simulink model "time_delay_continuous_model"  (R2023b)
settings: Solver=VariableStepAuto  StartTime=0.0  StopTime=20  RelTol=1e-3
values from neighbouring files (symbols this model uses):
  A = [Aaa Aab; Aba Abb]    [compensated_minimum_order_controller.m]    (also in compensated_observer_controller.m = [A Bv*Cc; zeros(1, 3) Ac]; direct_comp_calib.m; direct_compensated_minimum_order_controller.m; experiment_calc.m)
  AA = [A-Bv*K Bv*(Kb-[0 1 0]*A_b*kc); zeros(2, 3) Ae-Ko*Aab]    [compensated_minimum_order_controller.m]    (also in compensated_observer_controller.m = [A-Bv*K Bv*K; zeros(4) A-Ke*C]; direct_comp_calib.m = [A-Bv*K Bv*Kb; zeros(2, 3) Abb-Ko*Aab]; direct_compensated_minimum_order_controller.m = [A-Bv*K Bv*Kb; zeros(2, 3) Abb-Ko*Aab]; experiment_calc.m = [A-Bv*K Bv*Kb; zeros([2, 3]) Abb - Ko*Aab])
  Ahat = Abb - Ko*Aab    [experiment_calc.m]    (also in experiment_sym.m; simple_time_delay_discrete.m; simple_time_delay_sym.m; time_delay_continuous.m)
  Aimp = [0 1; -Ke/Me -Be/Me]    [experiment_calc.m]    (also in experiment_sym.m; time_delay_continuous.m; time_delay_continuous_sym.m; time_delay_discrete.m)
  Atilde = Ahat - Fhat_v*Kb    [experiment_calc.m]    (also in experiment_sym.m; simple_time_delay_discrete.m = Ahat - Fhat*Kb; simple_time_delay_sym.m = Ahat - Fhat*Kb; time_delay_continuous.m)
  B = -8*P.*M*0.05    [comp_controller_param_map.m]    (also in compensated_minimum_order_controller.m = [Bt Bv]; compensated_observer_controller.m = [0 0; 1/J 0; 0 1/L]; direct_comp_calib.m = [Bt Bv]; direct_compensated_minimum_order_controller.m = [Bt Bv])
  BB = [Bt - Bv*kc; zeros(2, 1)]    [compensated_minimum_order_controller.m]    (also in compensated_observer_controller.m = [Bt; Bt]; direct_comp_calib.m; direct_compensated_minimum_order_controller.m; experiment_calc.m = [Bv*Ka Bt - Bv*kc; zeros([2, 2])])
  Bhat = Ahat*Ko + Aba - Ko*Aaa    [experiment_calc.m]    (also in experiment_sym.m; simple_time_delay_discrete.m; simple_time_delay_sym.m; time_delay_continuous.m)
  Bimp = [0 0; Ke/Me 1/Me]    [experiment_calc.m]    (also in experiment_sym.m; time_delay_continuous.m; time_delay_continuous_sym.m; time_delay_discrete.m)
  Btilde = [Btilde_r Btilde_tau Btilde_y]    [experiment_calc.m]    (also in experiment_sym.m; simple_time_delay_discrete.m = [Btilde_r Btilde_y]; simple_time_delay_sym.m = [Btilde_r Btilde_y]; time_delay_continuous.m)
  C = [1 0 0]    [compensated_minimum_order_controller.m]    (also in compensated_observer_controller.m = [C 0]; direct_comp_calib.m; direct_compensated_minimum_order_controller.m; experiment_calc.m)
  CC = eye(5)    [compensated_minimum_order_controller.m]    (also in compensated_observer_controller.m = eye(8); direct_comp_calib.m; direct_compensated_minimum_order_controller.m; experiment_calc.m)
  Chat = [zeros([1, 2]); eye(2)]    [experiment_calc.m]    (also in experiment_sym.m; simple_time_delay_discrete.m = [0; 1]; simple_time_delay_sym.m = [0; 1]; time_delay_continuous.m)
  Cimp = [1 0]    [experiment_calc.m]    (also in experiment_sym.m = eye(2); time_delay_continuous.m = eye(2); time_delay_continuous_sym.m; time_delay_discrete.m = eye(2))
  Ctilde = -Kb    [experiment_calc.m]    (also in experiment_sym.m; simple_time_delay_discrete.m; simple_time_delay_sym.m; time_delay_continuous.m)
  D = [0 0]    [compensated_minimum_order_controller.m]    (also in compensated_observer_controller.m = 0; direct_comp_calib.m; direct_compensated_minimum_order_controller.m; experiment_calc.m)
  DD = zeros(5, 1)    [compensated_minimum_order_controller.m]    (also in compensated_observer_controller.m = zeros(8, 1); direct_comp_calib.m; direct_compensated_minimum_order_controller.m; experiment_calc.m = zeros([5, 2]))
  Dhat = [1; Ko]    [experiment_calc.m]    (also in experiment_sym.m; simple_time_delay_discrete.m; simple_time_delay_sym.m; time_delay_continuous.m)
  Dimp = zeros(2)    [experiment_calc.m]    (also in experiment_sym.m; time_delay_continuous.m; time_delay_continuous_sym.m; time_delay_discrete.m)
  Dtilde = [Ka -kc -(Ka + Kb*Ko)]    [experiment_calc.m]    (also in experiment_sym.m; simple_time_delay_discrete.m = [Ka -(Ka + Kb*Ko)]; simple_time_delay_sym.m = [Ka -(Ka + Kb*Ko)]; time_delay_continuous.m)
  ei = [0; 0]    [experiment_sym.m]    (also in simple_time_delay_discrete.m = 0; time_delay_continuous.m; time_delay_discrete.m; time_delay_discrete_fourier.m)
  Fhat_tau = Btb - Ko*Bta    [experiment_calc.m]    (also in experiment_sym.m; time_delay_continuous.m; time_delay_continuous_sym.m; time_delay_discrete.m)
  Fhat_v = Bvb - Ko*Bva    [experiment_calc.m]    (also in experiment_sym.m; time_delay_continuous.m; time_delay_continuous_sym.m; time_delay_discrete.m)
  K = place(A, Bv, P)    [compensated_minimum_order_controller.m]    (also in compensated_observer_controller.m; direct_comp_calib.m = acker(A, Bv, P); direct_compensated_minimum_order_controller.m = acker(A, Bv, P); experiment_calc.m = [0 0 1]/Cm*pd)
  Ka = K(1)    [compensated_minimum_order_controller.m]    (also in direct_comp_calib.m; direct_compensated_minimum_order_controller.m; experiment_calc.m; experiment_sym.m)
  kc = (R+K(3))/Km-Ka/Ke    [compensated_minimum_order_controller.m]    (also in direct_comp_calib.m; direct_compensated_minimum_order_controller.m; experiment_calc.m; experiment_sym.m)
  nutildei = nui - ei    [experiment_sym.m]    (also in simple_time_delay_discrete.m; time_delay_continuous.m; time_delay_discrete.m)
  xi = [1; 0; 0]    [experiment_sym.m]    (also in simple_time_delay_discrete.m = [1; 0]; time_delay_continuous.m = [0; 0; 0]; time_delay_discrete.m = [0; 0; 0]; time_delay_discrete_fourier.m)
settings Model: Creator=tamas  LastModifiedBy=tamas

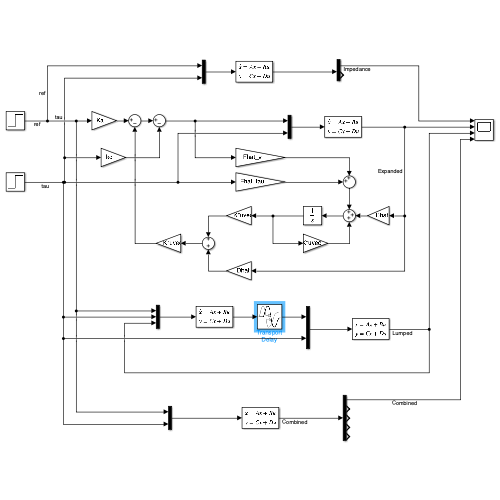
[thumbnail: Simulink's stored preview of the top-level diagram]
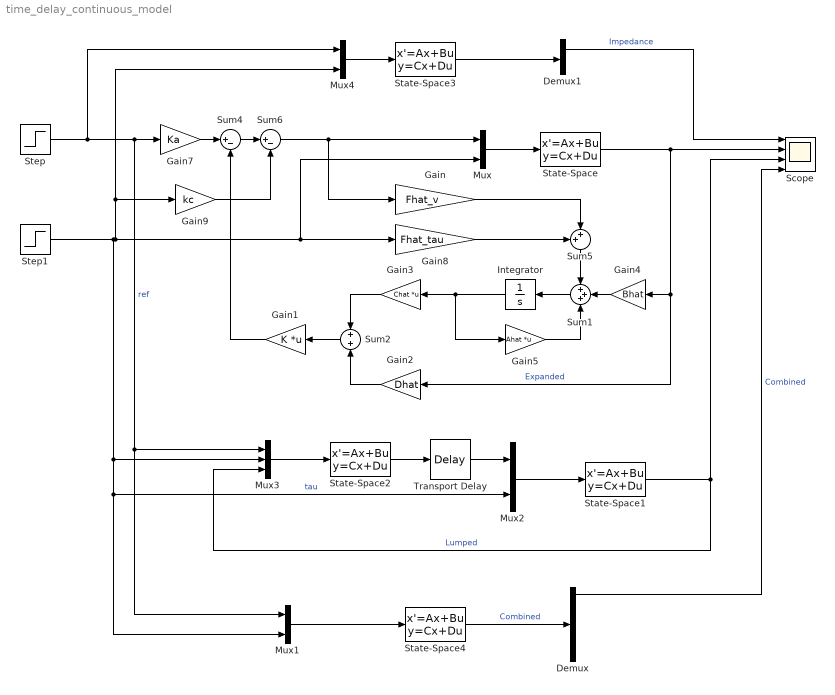
== system time_delay_continuous_model ==
  Demux : Demux  Outputs=5
  Demux1 : Demux  Outputs=2
  Gain : Gain  Gain=Fhat_v
  Gain1 : Gain  Gain=K  Multiplication=Matrix(K*u) (u vector)
  Gain2 : Gain  Gain=Dhat
  Gain3 : Gain  Gain=Chat  Multiplication=Matrix(K*u) (u vector)
  Gain4 : Gain  Gain=Bhat
  Gain5 : Gain  Gain=Ahat  Multiplication=Matrix(K*u) (u vector)
  Gain7 : Gain  Gain=Ka
  Gain8 : Gain  Gain=Fhat_tau
  Gain9 : Gain  Gain=kc
  Integrator : Integrator  InitialCondition=nutildei
  Mux{,1..2,4} (4 alike) : Mux  Inputs=2
  Mux3 : Mux  Inputs=3
  Scope : Scope  NumInputPorts=4
  State-Space : StateSpace  A=A  B=B  C=C  D=D  InitialCondition=xi
  State-Space1 : StateSpace  A=A  B=B  C=C  D=D  InitialCondition=xi
  State-Space2 : StateSpace  A=Atilde  B=Btilde  C=Ctilde  D=Dtilde  InitialCondition=nutildei
  State-Space3 : StateSpace  A=Aimp  B=Bimp  C=Cimp  D=Dimp  InitialCondition=xi(1:2)
  State-Space4 : StateSpace  A=AA  B=BB  C=CC  D=DD  InitialCondition=[xi; ei]
  Step : Step  Time=0  After=0  SampleTime=0
  Step1 : Step  Time=0  SampleTime=0
  Sum1 : Sum  Inputs=+++
  Sum2 : Sum  Inputs=+|+
  Sum4 : Sum  Inputs=|+-
  Sum5 : Sum  Inputs=++|
  Sum6 : Sum  Inputs=|+-
  Transport Delay : TransportDelay  DelayTime=0
  wires:
  State-Space/1 -> Gain4/1, Gain2/1, Scope/2  "Expanded"
  Gain1/1 -> Sum4/2
  Gain4/1 -> Sum1/2
  Sum1/1 -> Integrator/1
  Integrator/1 -> Gain5/1, Gain3/1
  Gain3/1 -> Sum2/1
  Gain2/1 -> Sum2/2
  Sum2/1 -> Gain1/1
  Gain5/1 -> Sum1/3
  State-Space1/1 -> Scope/3, Mux3/3  "Lumped"
  Demux/1 -> Scope/4  "Combined"
  Sum6/1 -> Gain/1, Mux/1
  Gain7/1 -> Sum4/1
  Mux/1 -> State-Space/1
  Sum5/1 -> Sum1/1
  Gain/1 -> Sum5/2
  Gain8/1 -> Sum5/1
  Mux1/1 -> State-Space4/1
  Mux2/1 -> State-Space1/1
  Mux3/1 -> State-Space2/1
  State-Space4/1 -> Demux/1  "Combined"
  Sum4/1 -> Sum6/1
  Gain9/1 -> Sum6/2
  Mux4/1 -> State-Space3/1
  Step1/1 -> Mux1/2, Mux2/2, Mux3/2, Mux4/2, Gain9/1, Mux/2, Gain8/1  "tau"
  Step/1 -> Mux1/1, Mux3/1, Gain7/1, Mux4/1  "ref"
  State-Space3/1 -> Demux1/1
  Demux1/1 -> Scope/1  "Impedance"
  Transport Delay/1 -> Mux2/1
  State-Space2/1 -> Transport Delay/1
